simulink model "synapse"  (Simulink 8.3)
settings: Solver=ode45  StartTime=0.0  StopTime=2  MaxStep=1e-3  RelTol=1e-3
values from neighbouring files (symbols this model uses):
  tau = 0.02    [test_synapse.m]
  v0 = 1    [test_synapse.m]
  wei = 0.1    [test_synapse.m]
undefined symbols (not defined in the file): fun_type
settings Model: Creator=wjj  LastModifiedBy=wjj
settings DataIOCC: SignalLoggingSaveFormat=Dataset
settings DebuggingCC: UnderspecifiedInitializationDetection=Simplified  StateNameClashWarn=none
settings GRTTargetCC: CombineOutputUpdateFcns=on  GRTInterface=off

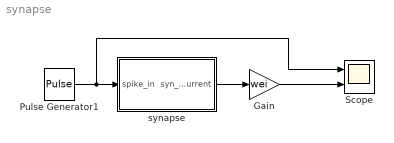
== system synapse ==
  Gain : Gain  Gain=wei
  Pulse Generator1 : DiscretePulseGenerator  PulseType=Time based  Period=1  PulseWidth=0.5  PhaseDelay=0.1
  Scope : Scope  NumInputPorts=2
      settings: YMin=-5~-0.1  YMax=5~0.6
  synapse : Subsystem  mask{v0=v0, tau=tau, fun_type=fun_type}
  wires:
  Pulse Generator1/1 -> synapse/1(spike_in), Scope/1
  synapse/1(syn_current) -> Gain/1
  Gain/1 -> Scope/2

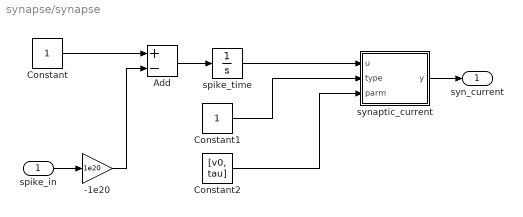
== system synapse/synapse ==
  spike_in : Inport
  -1e20 : Gain  Gain=1e20
  Add : Sum  Inputs=+-
  Constant : Constant
  Constant1 : Constant
  Constant2 : Constant  Value=[v0, tau]
  spike_time : Integrator  InitialCondition=10  LimitOutput=on  UpperSaturationLimit=10  LowerSaturationLimit=0
  synaptic_current : MATLAB Function  TreatAsAtomicUnit=on
  syn_current : Outport
  wires:
  Add/1 -> spike_time/1
  spike_time/1 -> synaptic_current/1(u)
  Constant1/1 -> synaptic_current/2(type)
  synaptic_current/1(y) -> syn_current/1
  -1e20/1 -> Add/2
  Constant/1 -> Add/1
  Constant2/1 -> synaptic_current/3(parm)
  spike_in/1 -> -1e20/1

== matlab function synapse/synaptic_current ==
  data: u input double; y output double; type input double; parm input double
function y = sf(u, type, parm)
%#codegen
v0 = parm(1);
tau = parm(2);
if type == 0
    y = v0*exp(-u/tau);
elseif type == 1;
    y = v0*exp(1)*(u/tau)*exp(-u/tau);
else
    y = 0;
end
